simulink model "p7"  (R2021b)
settings: Solver=VariableStepAuto  StartTime=0.0  StopTime=30  RelTol=1e-3
settings Model: Creator=mahya  LastModifiedBy=mahya

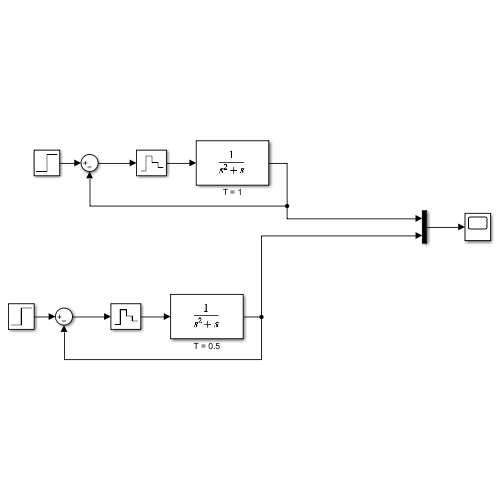
[thumbnail: Simulink's stored preview of the top-level diagram]
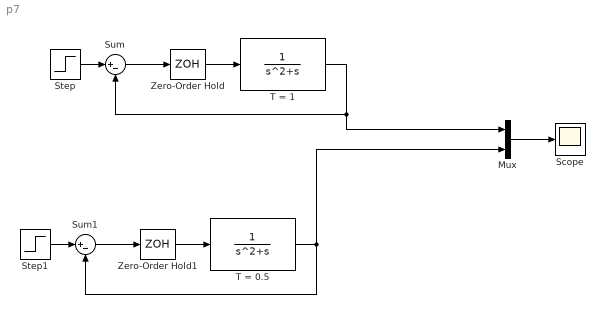
== system p7 ==
  Mux : Mux  Inputs=2
  Scope : Scope
  Step : Step  Time=0  SampleTime=0
  Step1 : Step  Time=0  SampleTime=0
  Sum : Sum  Inputs=|+-
  Sum1 : Sum  Inputs=|+-
  T = 0.5 : TransferFcn  Denominator=[1 1 0]
  T = 1 : TransferFcn  Denominator=[1 1 0]
  Zero-Order Hold : ZeroOrderHold
  Zero-Order Hold1 : ZeroOrderHold  SampleTime=0.5
  wires:
  Zero-Order Hold/1 -> T = 1/1
  Zero-Order Hold1/1 -> T = 0.5/1
  Sum1/1 -> Zero-Order Hold1/1
  T = 1/1 -> Mux/1, Sum/2
  Step/1 -> Sum/1
  Sum/1 -> Zero-Order Hold/1
  Step1/1 -> Sum1/1
  T = 0.5/1 -> Sum1/2, Mux/2
  Mux/1 -> Scope/1
